simulink model "Q61"  (R2026a)
settings: Solver=VariableStepAuto
values from neighbouring files (symbols this model uses):
  m = 'Q2_Van_der_Pol'; fresh(m,'30')    [complete_assignment.m]
  s = sim(m)    [complete_assignment.m]
  T3 = feedback(C3*G3,1)    [complete_assignment.m]
  T4 = feedback(C4*G4,1)    [complete_assignment.m]
undefined symbols (not defined in the file or in its folder): d4_0, d4_f, H, Kd1, Kd2, Kd3, Kd4, Ki1, Ki2, Ki3, Ki4, Kp1, Kp2, Kp3, Kp4, L1, L2, L3, L4, m4, q1_0, q1_f, q2_0, q2_f, q3_0, q3_f, T1, T2, ts1, ts2, ts3, ts4, W, X, Y, Z
libraries: sm_lib x32, nesl_utility x10, slpidlib x4
(part 2 of 2)

== matlab function Q61/R2_Trajectory ==
  data: t input; q2d output; q2_0 parameter; q2_f parameter; T2 parameter; ts2 parameter
function q2d = fcn(t, q2_0, q2_f, T2, ts2)
% R2_Trajectory
% ---------------------------------------------------------
% 功能：
%   生成 RRRP 机械臂第 2 个转动关节 R2 的期望角度轨迹。
%
% 输入：
%   t     - 当前仿真时间，单位：s
%   q2_0  - R2 初始关节角，单位：rad
%   q2_f  - R2 目标关节角，单位：rad
%   T2    - R2 完成运动所需的持续时间，单位：s
%   ts2   - R2 开始运动的时刻，单位：s
%
% 输出：
%   q2d   - R2 在当前时刻的期望关节角，单位：rad
%
% 本模块使用五次多项式时间标度，使 R2 从初始角度
% 平滑运动到目标角度，并保证起止速度和加速度为 0。
% ---------------------------------------------------------

% R2 初始角度
q0 = q2_0;

% R2 目标角度
qf = q2_f;

% R2 开始运动时间
ts = ts2;

% R2 运动持续时间
T = T2;


% ---------- 阶段 1：保持初始位置 ----------
if t <= ts

    % 尚未到达 R2 的启动时刻
    q2d = q0;


% ---------- 阶段 2：执行五次多项式轨迹 ----------
elseif t < ts + T

    % 时间归一化
    % 将 [ts, ts+T] 映射到 [0,1]
    s = (t - ts)/T;

    % 五次多项式时间标度
    h = 10*s^3 - 15*s^4 + 6*s^5;

    % 根据 h 从初始角度平滑过渡至目标角度
    q2d = q0 + (qf - q0)*h;


% ---------- 阶段 3：保持最终目标 ----------
else

    q2d = qf;

end

== matlab function Q61/R3_Trajectory ==
  data: t input; q3d output; q3_0 parameter; q3_f parameter; T3 parameter; ts3 parameter
function q3d = fcn(t, q3_0, q3_f, T3, ts3)
% R3_Trajectory
% ---------------------------------------------------------
% 功能：
%   生成 RRRP 机械臂第 3 个转动关节 R3 的期望角度轨迹。
%
% 输入：
%   t     - 当前仿真时间，单位：s
%   q3_0  - R3 初始关节角，单位：rad
%   q3_f  - R3 目标关节角，单位：rad
%   T3    - R3 完成运动所需的持续时间，单位：s
%   ts3   - R3 开始运动的时刻，单位：s
%
% 输出：
%   q3d   - R3 在当前时刻的期望关节角，单位：rad
%
% 采用五次多项式时间标度，使 R3 的位置、速度及
% 加速度在起始和结束位置具有良好的连续性。
% ---------------------------------------------------------

% R3 初始角度
q0 = q3_0;

% R3 最终目标角度
qf = q3_f;

% R3 开始执行运动的时间
ts = ts3;

% R3 从起点到终点所需时间
T = T3;


% ---------- 阶段 1：运动开始前 ----------
if t <= ts

    % 保持 R3 初始位置
    q3d = q0;


% ---------- 阶段 2：平滑运动 ----------
elseif t < ts + T

    % 将实际时间转换为 0~1 的归一化时间
    s = (t - ts)/T;

    % 五次多项式时间标度函数
    h = 10*s^3 - 15*s^4 + 6*s^5;

    % 当前 R3 期望角度
    q3d = q0 + (qf - q0)*h;


% ---------- 阶段 3：运动完成 ----------
else

    % 保持最终目标角度
    q3d = qf;

end
